simulink model "ASRAM"  (R2021b)
settings: Solver=VariableStepAuto  StartTime=0.0  StopTime=50  RelTol=1e-3
libraries: hdlsllib x5
settings Model: Creator=abhig  LastModifiedBy=abhig
settings DebuggingCC: UnconnectedInputMsg=none  UnconnectedOutputMsg=none  UnconnectedLineMsg=none
settings RTWCC: DLArmComputeVersion=20.02.1

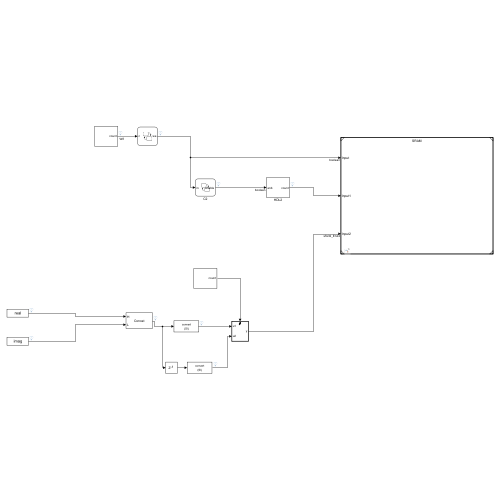
[thumbnail: Simulink's stored preview of the top-level diagram]
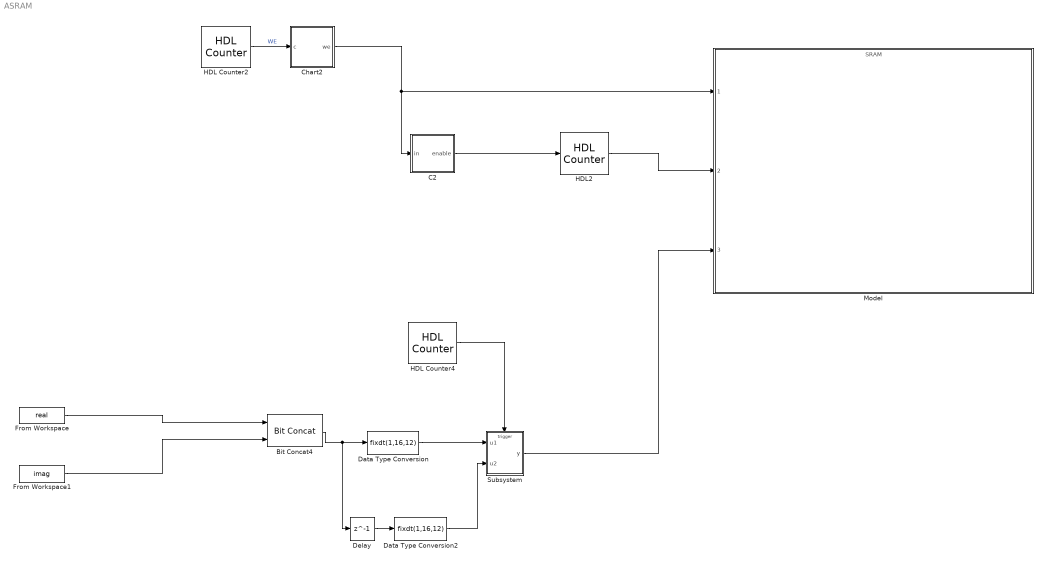
== system ASRAM ==
  Bit Concat4 : hdlsllib/Logic and Bit Operations/Bit Concat  numInputs=2
  C2 : Stateflow chart  TreatAsAtomicUnit=on
  Chart2 : Stateflow chart  TreatAsAtomicUnit=on
  Data Type Conversion : DataTypeConversion  OutDataTypeStr=fixdt(1,16,12)  ConvertRealWorld=Stored Integer (SI)
  Data Type Conversion2 : DataTypeConversion  OutDataTypeStr=fixdt(1,16,12)  ConvertRealWorld=Stored Integer (SI)
  Delay : Delay  DelayLength=1
  From Workspace : FromWorkspace  VariableName=real  SampleTime=1/t  Interpolate=off  OutputAfterFinalValue=Holding final value
  From Workspace1 : FromWorkspace  VariableName=imag  SampleTime=1/t  Interpolate=off  OutputAfterFinalValue=Holding final value
  HDL Counter2 : hdlsllib/Sources/HDL Counter  CountType=Count limited  CountInit=1  CountStep=1  CountMax=10  CountFromType=Initial value  CountFrom=1  CountResetPort=off  CountLoadPort=off  CountEnbPort=off  CountDirPort=off  CountHitOutputPort=off  CountDataType=Unsigned  CountWordLen=8  CountFracLen=0  CountSampTime=1
  HDL Counter4 : hdlsllib/Sources/HDL Counter  CountType=Count limited  CountInit=0  CountStep=1  CountMax=1  CountFromType=Initial value  CountFrom=0  CountResetPort=off  CountLoadPort=off  CountEnbPort=off  CountDirPort=off  CountHitOutputPort=off  CountDataType=Unsigned  CountWordLen=8  CountFracLen=0  CountSampTime=1
  HDL2 : hdlsllib/Sources/HDL Counter  CountType=Count limited  CountInit=1  CountStep=1  CountMax=10  CountFromType=Initial value  CountFrom=1  CountResetPort=off  CountLoadPort=off  CountEnbPort=on  CountDirPort=off  CountHitOutputPort=off  CountDataType=Unsigned  CountWordLen=8  CountFracLen=0  CountSampTime=1
  Model : ModelReference  ModelNameDialog=SRAM.slx  SimulationMode=Normal  ModelReferenceVersion=1.50
  Subsystem : Subsystem
  wires:
  Chart2/1(we) -> C2/1(in), Model/1
  Subsystem/1(y) -> Model/3
  From Workspace1/1 -> Bit Concat4/2
  Delay/1 -> Data Type Conversion2/1
  From Workspace/1 -> Bit Concat4/1
  HDL Counter4/1 -> Subsystem/Trigger
  Bit Concat4/1 -> Data Type Conversion/1, Delay/1
  C2/1(enable) -> HDL2/1
  HDL Counter2/1 -> Chart2/1(c)  "WE"
  HDL2/1 -> Model/2
  Data Type Conversion/1 -> Subsystem/1(u1)
  Data Type Conversion2/1 -> Subsystem/2(u2)

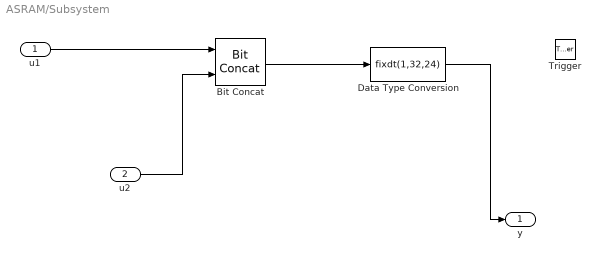
== system ASRAM/Subsystem ==
  u1 : Inport
  u2 : Inport  Port=2
  Trigger : TriggerPort  VariantControl=(inherit)  PortDimensions=1
  Bit Concat : hdlsllib/Logic and Bit Operations/Bit Concat  numInputs=2
  Data Type Conversion : DataTypeConversion  OutDataTypeStr=fixdt(1,32,24)  ConvertRealWorld=Stored Integer (SI)
  y : Outport
  wires:
  u2/1 -> Bit Concat/2
  u1/1 -> Bit Concat/1
  Bit Concat/1 -> Data Type Conversion/1
  Data Type Conversion/1 -> y/1

== stateflow chart ASRAM/C2 ==
  state default
    enable=true
  state add
    entry:x=0,enable=false;
    during :x=x+0.25;
  state x
    enable=false
  add -> x [order 2] : [in==0]
  (default) -> add
  default -> add [order 1] : [in==1]
  x -> add : [in==0]
  default -> x [order 2] : [in==1]
  add -> default [order 1] : [x>=0&&in==1]
  data: x local; enable output; in input

== stateflow chart ASRAM/Chart2 ==
  state d
    we=true
  state f
    we=true;
  state j
    we=false;
  state j1
    we=false;
  d -> d [order 2] : [c>=2&&c<=10]
  f -> f [order 1] : [c>=2&&c<=10]
  (default) -> d
  d -> f [order 1] : [c==1]
  f -> j1 [order 2] : [c==1]
  j -> d [order 2] : [c==1]
  j1 -> j [order 2] : [c==1]
  j -> j [order 1] : [c>=2 && c<=10]
  j1 -> j1 [order 1] : [c>=2 && c<10]
  data: c input; we output
